simulink model "Grue_NL_corrL"  (R2018b)
settings: Solver=ode45  StartTime=0.0  StopTime=dt  FixedStep=1e-4  RelTol=1e-3  EnableMultiTasking=on
values from neighbouring files (symbols this model uses):
  b = 0.4    [Ini_Grue.m]
  C0 = m*g*b    (= 2000)    [Ini_Grue.m]
  Cd = 20    [Ini_Grue.m]
  Cr = 20    [Ini_Grue.m]    (also in plot_things.m = Cr*kc)
  D = 0    [Ini_Grue.m]
  eta = -1/(C_1*(A-B*K)^-1*B_1)    [Ini_Grue.m]
  F = 0    [Ini_Grue.m]
  g = 10    [Ini_Grue.m]
  J = 50    [Ini_Grue.m]
  K = place(A,B,p)    [Ini_Grue.m]
  m = 500    [Ini_Grue.m]    (also in plot_things.m)
  Mc = 5000    [Ini_Grue.m]
  R = 15    [Ini_Grue.m]
  Ti = 5e-4    (= 0.0005)    [plot_things.m]
settings Model: Creator=abbasturki  LastModifiedBy=pac
settings DataIOCC: LimitDataPoints=on  SaveFormat=Array  SignalLoggingSaveFormat=ModelDataLogs
settings OptimizationCC: ExpressionDepthLimit=2147483647  LifeSpan=inf
settings DebuggingCC: UnderspecifiedInitializationDetection=Classic  MergeDetectMultiDrivingBlocksExec=none  SolverPrmCheckMsg=warning  FcnCallInpInsideContextMsg=warning  StateNameClashWarn=warning  SFUnexpectedBacktrackingDiag=warning  SFNoUnconditionalDefaultTransitionDiag=warning  SFExecutionAtInitializationDiag=none
settings HardwareCC: ProdBitPerPointer=32  ProdBitPerSizeT=32  ProdBitPerPtrDiffT=32  ProdLargestAtomicFloat=None  ProdIntDivRoundTo=Undefined  ProdEndianess=Unspecified  ProdWordSize=32  ProdHWDeviceType=32-bit Generic
settings ModelReferenceCC: PropagateSignalLabelsOutOfModel=off
settings SFSimCC: SimUseLocalCustomCode=off
settings RTWCC: RTWUseLocalCustomCode=off
settings CodeAppCC: StateflowObjectComments=on
settings GRTTargetCC: TargetLangStandard=C89/C90 (ANSI)  GeneratePreprocessorConditionals=Disable all  CombineOutputUpdateFcns=off  GRTInterface=on
settings ConfigComp: CovMetricSettings=dw  CovHtmlReporting=on  CovSaveCumulativeToWorkspaceVar=on  CovSaveSingleToWorkspaceVar=on  CovExternalEMLEnable=off

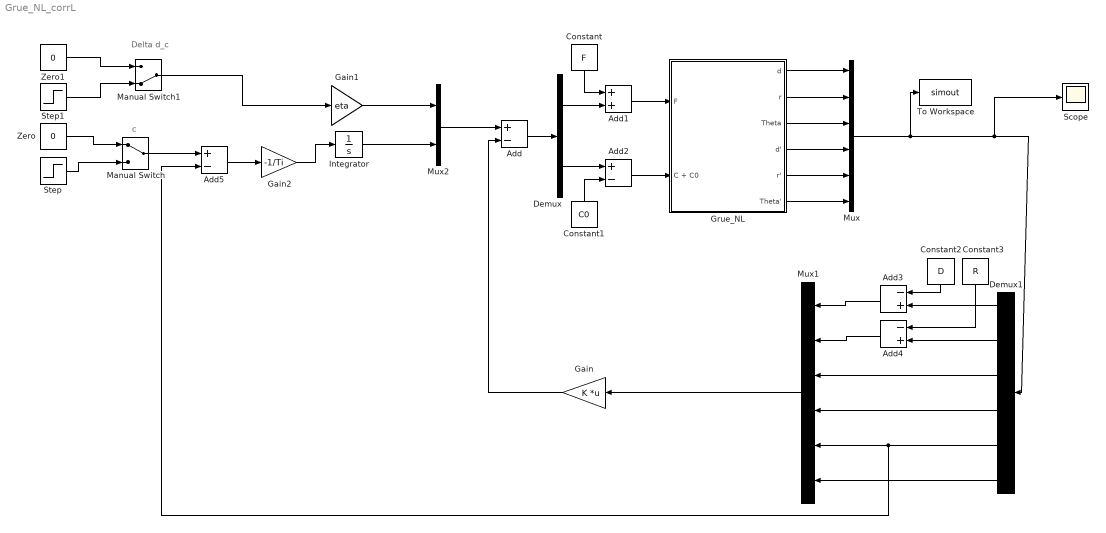
== system Grue_NL_corrL ==
  note: Delta d_c
  note: c
  Add : Sum  Inputs=+-
  Add1 : Sum
  Add2 : Sum  Inputs=+-
  Add3 : Sum  Inputs=-+
  Add4 : Sum  Inputs=-+
  Add5 : Sum  Inputs=+-
  Constant : Constant  Value=F
  Constant1 : Constant  Value=C0
  Constant2 : Constant  Value=D
  Constant3 : Constant  Value=R
  Demux : Demux  Outputs=2
  Demux1 : Demux  Outputs=6
  Gain : Gain  Gain=K  Multiplication=Matrix(K*u) (u vector)
  Gain1 : Gain  Gain=eta
  Gain2 : Gain  Gain=-1/Ti
  Grue_NL : Subsystem
  Integrator : Integrator
  Manual Switch : ManualSwitch
  Manual Switch1 : ManualSwitch  CurrentSetting=0
  Mux : Mux  Inputs=6
  Mux1 : Mux  Inputs=6
  Mux2 : Mux  Inputs=2
  Scope : Scope
  Step : Step  SampleTime=0
  Step1 : Step  After=100  SampleTime=0
  To Workspace : ToWorkspace  VariableName=simout  SaveFormat=Timeseries  SampleTime=-1
  Zero : Constant  Value=0  OutDataTypeStr=Inherit: Inherit via back propagation
  Zero1 : Constant  Value=0  OutDataTypeStr=Inherit: Inherit via back propagation
  wires:
  Grue_NL/1(d) -> Mux/1
  Grue_NL/2(r) -> Mux/2
  Grue_NL/3(Theta) -> Mux/3
  Grue_NL/4(d') -> Mux/4
  Grue_NL/5(r') -> Mux/5
  Grue_NL/6(Theta') -> Mux/6
  Add/1 -> Demux/1
  Gain/1 -> Add/2
  Add1/1 -> Grue_NL/1(F)
  Demux/1 -> Add1/2
  Add2/1 -> Grue_NL/2(C + C0)
  Constant/1 -> Add1/1
  Constant1/1 -> Add2/2
  Demux/2 -> Add2/1
  Mux1/1 -> Gain/1
  Demux1/1 -> Add3/2
  Constant2/1 -> Add3/1
  Add3/1 -> Mux1/1
  Demux1/2 -> Add4/2
  Add4/1 -> Mux1/2
  Constant3/1 -> Add4/1
  Demux1/3 -> Mux1/3
  Demux1/4 -> Mux1/4
  Demux1/5 -> Add5/2, Mux1/5
  Demux1/6 -> Mux1/6
  Integrator/1 -> Mux2/2
  Gain2/1 -> Integrator/1
  Step/1 -> Manual Switch/2
  Zero1/1 -> Manual Switch1/1
  Step1/1 -> Manual Switch1/2
  Manual Switch1/1 -> Gain1/1
  Zero/1 -> Manual Switch/1
  Manual Switch/1 -> Add5/1
  Add5/1 -> Gain2/1
  Gain1/1 -> Mux2/1
  Mux2/1 -> Add/1
  Mux/1 -> To Workspace/1, Scope/1, Demux1/1

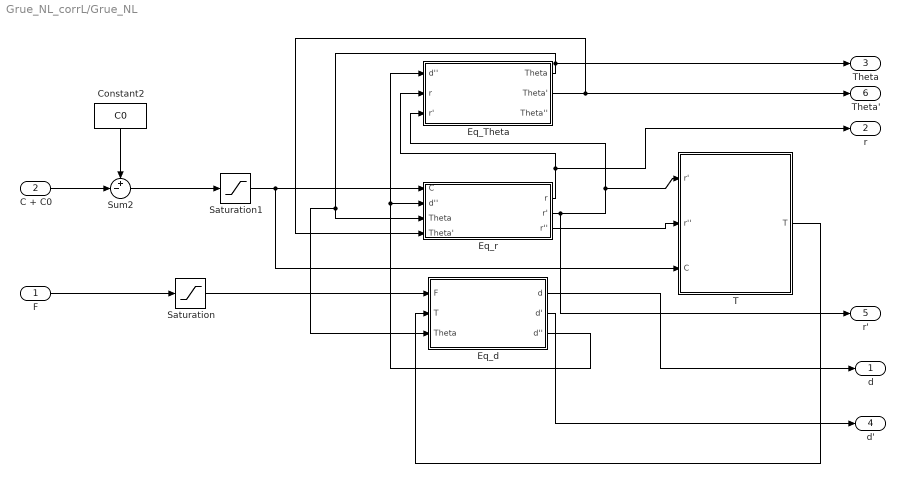
== system Grue_NL_corrL/Grue_NL ==
  F : Inport
  C + C0 : Inport  Port=2
  Constant2 : Constant  Value=C0
  Eq_Theta : Subsystem
  Eq_d : Subsystem
  Eq_r : Subsystem
  Saturation : Saturate  UpperLimit=1e4  LowerLimit=-1e4
  Saturation1 : Saturate  UpperLimit=3e3  LowerLimit=-3e3
  Sum2 : Sum  Inputs=+-|
  T : Subsystem
  d : Outport
  r : Outport  Port=2
  Theta : Outport  Port=3
  d' : Outport  Port=4
  r' : Outport  Port=5
  Theta' : Outport  Port=6
  wires:
  Eq_r/2(r') -> Eq_Theta/3(r'), T/1(r'), r'/1
  Eq_r/1(r) -> Eq_Theta/2(r), r/1
  Eq_d/3(d'') -> Eq_Theta/1(d''), Eq_r/2(d'')
  Eq_d/2(d') -> d'/1
  Eq_Theta/1(Theta) -> Eq_d/3(Theta), Eq_r/3(Theta), Theta/1
  Eq_Theta/2(Theta') -> Eq_r/4(Theta'), Theta'/1
  Eq_r/3(r'') -> T/2(r'')
  F/1 -> Saturation/1
  T/1(T) -> Eq_d/2(T)
  Eq_d/1(d) -> d/1
  Saturation/1 -> Eq_d/1(F)
  Saturation1/1 -> Eq_r/1(C), T/3(C)
  Constant2/1 -> Sum2/1
  Sum2/1 -> Saturation1/1
  C + C0/1 -> Sum2/2

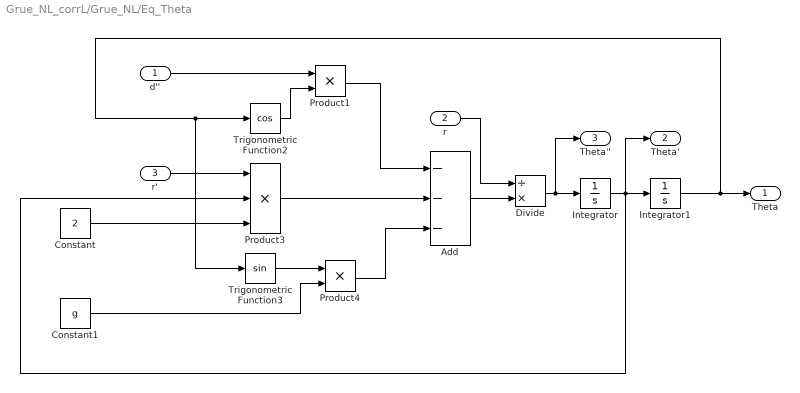
== system Grue_NL_corrL/Grue_NL/Eq_Theta ==
  d'' : Inport
  r : Inport  Port=2
  r' : Inport  Port=3
  Add : Sum  Inputs=---
  Constant : Constant  Value=2
  Constant1 : Constant  Value=g
  Divide : Product  Inputs=/*
  Integrator : Integrator
  Integrator1 : Integrator
  Product1 : Product  RndMeth=Zero
  Product3 : Product  Inputs=3  RndMeth=Zero
  Product4 : Product  RndMeth=Zero
  Trigonometric Function2 : Trigonometry  Operator=cos
  Trigonometric Function3 : Trigonometry
  Theta : Outport
  Theta' : Outport  Port=2
  Theta'' : Outport  Port=3
  wires:
  d''/1 -> Product1/1
  Trigonometric Function2/1 -> Product1/2
  r'/1 -> Product3/1
  Constant/1 -> Product3/3
  Trigonometric Function3/1 -> Product4/1
  Constant1/1 -> Product4/2
  Product1/1 -> Add/1
  Product3/1 -> Add/2
  Product4/1 -> Add/3
  r/1 -> Divide/1
  Add/1 -> Divide/2
  Divide/1 -> Integrator/1, Theta''/1
  Integrator/1 -> Integrator1/1, Product3/2, Theta'/1
  Integrator1/1 -> Theta/1, Trigonometric Function2/1, Trigonometric Function3/1

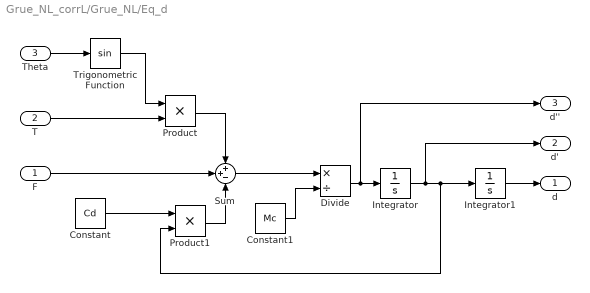
== system Grue_NL_corrL/Grue_NL/Eq_d ==
  F : Inport
  T : Inport  Port=2
  Theta : Inport  Port=3
  Constant : Constant  Value=Cd
  Constant1 : Constant  Value=Mc
  Divide : Product  Inputs=*/
  Integrator : Integrator
  Integrator1 : Integrator
  Product : Product  RndMeth=Zero
  Product1 : Product  RndMeth=Zero
  Sum : Sum  Inputs=++-
  Trigonometric Function : Trigonometry
  d : Outport
  d' : Outport  Port=2
  d'' : Outport  Port=3
  wires:
  Product/1 -> Sum/1
  Trigonometric Function/1 -> Product/1
  Product1/1 -> Sum/3
  Constant/1 -> Product1/1
  Sum/1 -> Divide/1
  Constant1/1 -> Divide/2
  Divide/1 -> Integrator/1, d''/1
  Integrator/1 -> Integrator1/1, Product1/2, d'/1
  F/1 -> Sum/2
  T/1 -> Product/2
  Theta/1 -> Trigonometric Function/1
  Integrator1/1 -> d/1

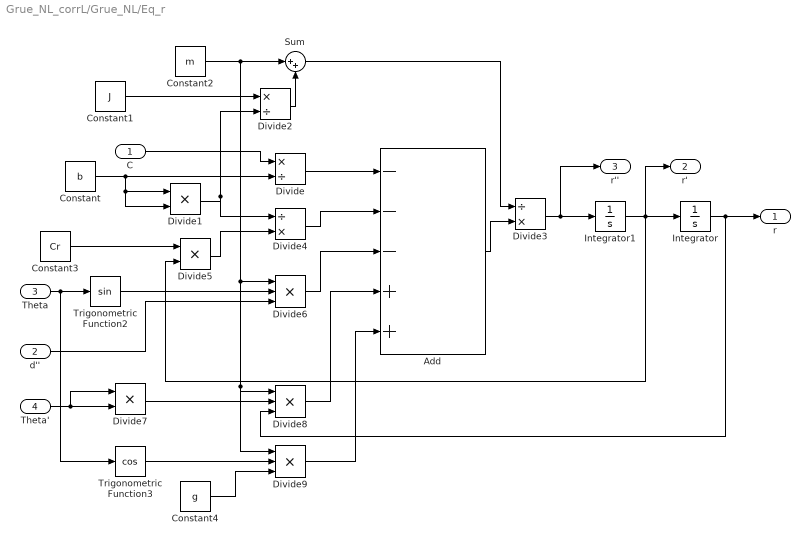
== system Grue_NL_corrL/Grue_NL/Eq_r ==
  C : Inport
  d'' : Inport  Port=2
  Theta : Inport  Port=3
  Theta' : Inport  Port=4
  Add : Sum  Inputs=---++
  Constant : Constant  Value=b
  Constant1 : Constant  Value=J
  Constant2 : Constant  Value=m
  Constant3 : Constant  Value=Cr
  Constant4 : Constant  Value=g
  Divide : Product  Inputs=*/
  Divide1 : Product  Inputs=**
  Divide2 : Product  Inputs=*/
  Divide3 : Product  Inputs=/*
  Divide4 : Product  Inputs=/*
  Divide5 : Product  Inputs=**
  Divide6 : Product  Inputs=***
  Divide7 : Product  Inputs=**
  Divide8 : Product  Inputs=***
  Divide9 : Product  Inputs=***
  Integrator : Integrator  InitialCondition=R
  Integrator1 : Integrator
  Sum : Sum  Inputs=|++
  Trigonometric Function2 : Trigonometry
  Trigonometric Function3 : Trigonometry  Operator=cos
  r : Outport
  r' : Outport  Port=2
  r'' : Outport  Port=3
  wires:
  C/1 -> Divide/1
  Constant/1 -> Divide/2, Divide1/1, Divide1/2
  Divide/1 -> Add/1
  Constant2/1 -> Sum/1, Divide6/1, Divide8/1, Divide9/1
  Divide2/1 -> Sum/2
  Constant1/1 -> Divide2/1
  Divide1/1 -> Divide2/2, Divide4/1
  Sum/1 -> Divide3/1
  Add/1 -> Divide3/2
  Divide3/1 -> Integrator1/1, r''/1
  Integrator1/1 -> Integrator/1, Divide5/2, r'/1
  Constant3/1 -> Divide5/1
  Divide5/1 -> Divide4/2
  Divide4/1 -> Add/2
  Theta/1 -> Trigonometric Function2/1, Trigonometric Function3/1
  d''/1 -> Divide6/3
  Trigonometric Function2/1 -> Divide6/2
  Divide6/1 -> Add/3
  Theta'/1 -> Divide7/2, Divide7/1
  Divide7/1 -> Divide8/2
  Integrator/1 -> Divide8/3, r/1
  Divide8/1 -> Add/4
  Trigonometric Function3/1 -> Divide9/2
  Constant4/1 -> Divide9/3
  Divide9/1 -> Add/5

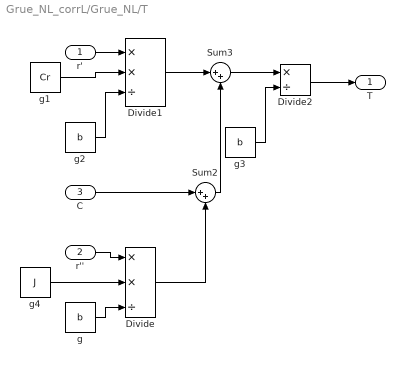
== system Grue_NL_corrL/Grue_NL/T ==
  r' : Inport
  r'' : Inport  Port=2
  C : Inport  Port=3
  Divide : Product  Inputs=**/
  Divide1 : Product  Inputs=**/
  Divide2 : Product  Inputs=*/
  Sum2 : Sum  Inputs=|++
  Sum3 : Sum  Inputs=|++
  g : Constant  Value=b
  g1 : Constant  Value=Cr
  g2 : Constant  Value=b
  g3 : Constant  Value=b
  g4 : Constant  Value=J
  T : Outport
  wires:
  r''/1 -> Divide/1
  C/1 -> Sum2/1
  Divide/1 -> Sum2/2
  r'/1 -> Divide1/1
  g1/1 -> Divide1/2
  g2/1 -> Divide1/3
  Divide1/1 -> Sum3/1
  Sum2/1 -> Sum3/2
  Sum3/1 -> Divide2/1
  g3/1 -> Divide2/2
  Divide2/1 -> T/1
  g/1 -> Divide/3
  g4/1 -> Divide/2
